simulink model "Ex6_2"  (Simulink 6.0)
settings: Solver=FixedStepDiscrete  SolverMode=SingleTasking  StartTime=0.0  StopTime=Ts*10  FixedStep=Ts  RelTol=1e-3  AbsTol=1e-6
values from neighbouring files (symbols this model uses):
  Ampl = 10^(Amp_dB/20)    (= 0.758577575029)    [Ex6_4Launch.m]
  finrad = Fin*2*pi    (= 28141.7979422)    [Ex6_4Launch.m]
  MultiBit = 1    [Ex6_4Launch.m]
  Ncomp = 1    [Ex6_4Launch.m]
  QuantSat = 0    [Ex6_4Launch.m]
  SatFirst = 1    [Ex6_4Launch.m]
  SatQuant = 0    [Ex6_4Launch.m]
  SatSecond = 1    [Ex6_4Launch.m]
  Ts = 1/Fs    (= 3.54308390023e-07)    [Ex6_4Launch.m]
  VrefN = -1    [Ex6_4Launch.m]
  VrefP = 1    [Ex6_4Launch.m]
  Vsat1 = 1.85    [Ex6_4Launch.m]
  Vsat2 = 2.5    [Ex6_4Launch.m]
undefined symbols (not defined in the file or in its folder): Quantiz
settings Model: Creator=francomaloberti  LastModifiedBy=Cri  ExtModeAutoUpdateStatusClock=off
settings DataIOCC: LimitDataPoints=off  SignalLoggingName=sigsOut
settings OptimizationCC: BooleanDataType=off  InlineInvariantSignals=off
settings DebuggingCC: SolverPrmCheckMsg=none
settings HardwareCC: TargetUnknown=on

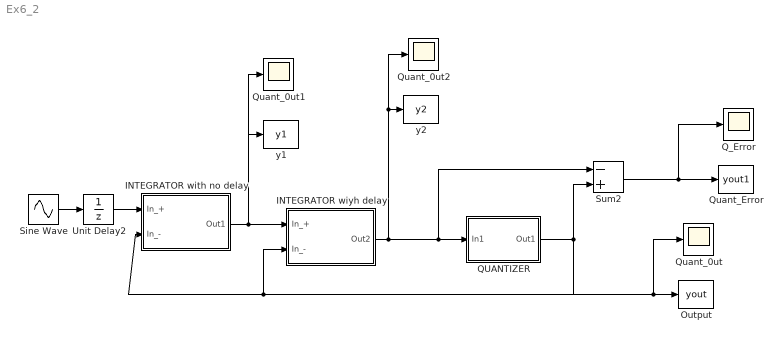
== system Ex6_2 ==
  INTEGRATOR with no delay : Subsystem
      mask Display:
      | patch([10 40 10 10], [0 20 40 0],[0 1 1])
      | plot([10 40 10 10], [0 20 40 0])
      | plot([0 10], [8 8])
      | plot([0 10], [28 28])
      | dpoly([1], [1 -1], 'z-')
      | port_label('input', 1, '+')
      | port_label('input', 2, '-')
  INTEGRATOR wiyh delay : Subsystem
      mask Display:
      | patch([10 40 10 10], [0 20 40 0],[1 0 1])
      | plot([10 40 10 10], [0 20 40 0])
      | plot([0 10], [8 8])
      | plot([0 10], [28 28])
      | dpoly([0 1], [1 -1], 'z-')
      | port_label('input', 1, '+')
      | port_label('input', 2, '-')
  Output : ToWorkspace  VariableName=yout  SampleTime=-1  SaveFormat=Array
  QUANTIZER : Subsystem
      mask Display:
      | plot([0 5 5 10 10 15 15], [0 0 5 5 10 10 15])
      | plot([25 30 30 35], [0 0 15 15])
      | disp('  or')
  Q_Error : Scope
      settings: SaveName=ScopeData2
  Quant_0ut : Scope
  Quant_0ut1 : Scope
  Quant_0ut2 : Scope
      settings: SaveName=ScopeData3
  Quant_Error : ToWorkspace  VariableName=yout1  SampleTime=-1  SaveFormat=Array
  Sine Wave : Sin  Amplitude=Ampl  Frequency=finrad  SampleTime=0
  Sum2 : Sum  Inputs=-+  SaturateOnIntegerOverflow=on  InputSameDT=on
  Unit Delay2 : UnitDelay  SampleTime=Ts
  y1 : ToWorkspace  VariableName=y1  SampleTime=-1  SaveFormat=Array
  y2 : ToWorkspace  VariableName=y2  SampleTime=-1  SaveFormat=Array
  wires:
  Sine Wave/1 -> Unit Delay2/1
  Unit Delay2/1 -> INTEGRATOR with no delay/1(In_+)
  INTEGRATOR wiyh delay/1(Out2) -> QUANTIZER/1(In1), Sum2/1, y2/1, Quant_0ut2/1
  INTEGRATOR with no delay/1(Out1) -> INTEGRATOR wiyh delay/1(In_+), y1/1, Quant_0ut1/1
  QUANTIZER/1(Out1) -> Sum2/2, INTEGRATOR wiyh delay/2(In_-), INTEGRATOR with no delay/2(In_-), Output/1, Quant_0ut/1
  Sum2/1 -> Q_Error/1, Quant_Error/1

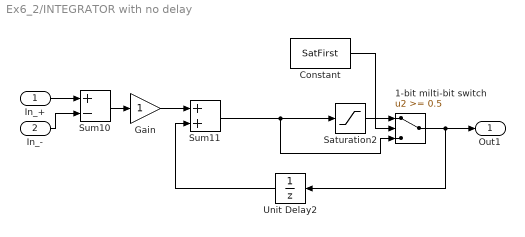
== system Ex6_2/INTEGRATOR with no delay ==
  In_+ : Inport  Port=1  LatchInput=off
  In_- : Inport  Port=2  LatchInput=off
  1-bit milti-bit switch : Switch  Threshold=0.5
  Constant : Constant  Value=SatFirst
  Gain : Gain  SaturateOnIntegerOverflow=on
  Saturation2 : Saturate  UpperLimit=Vsat1  LowerLimit=-Vsat1
  Sum10 : Sum  Inputs=+-  SaturateOnIntegerOverflow=on  InputSameDT=on
  Sum11 : Sum  SaturateOnIntegerOverflow=on  InputSameDT=on
  Unit Delay2 : UnitDelay  Orientation=left  SampleTime=Ts
  Out1 : Outport
  wires:
  Constant/1 -> 1-bit milti-bit switch/2
  1-bit milti-bit switch/1 -> Out1/1, Unit Delay2/1
  Saturation2/1 -> 1-bit milti-bit switch/1
  In_+/1 -> Sum10/1
  In_-/1 -> Sum10/2
  Sum11/1 -> 1-bit milti-bit switch/3, Saturation2/1
  Sum10/1 -> Gain/1
  Gain/1 -> Sum11/1
  Unit Delay2/1 -> Sum11/2

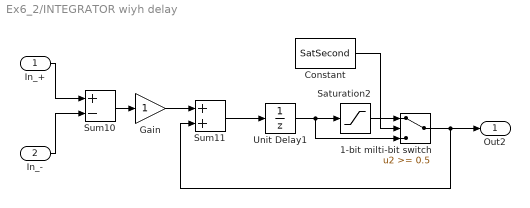
== system Ex6_2/INTEGRATOR wiyh delay ==
  In_+ : Inport  Port=1  LatchInput=off
  In_- : Inport  Port=2  LatchInput=off
  1-bit milti-bit switch : Switch  Threshold=0.5
  Constant : Constant  Value=SatSecond
  Gain : Gain  SaturateOnIntegerOverflow=on
  Saturation2 : Saturate  UpperLimit=Vsat2  LowerLimit=-Vsat2
  Sum10 : Sum  Inputs=+-  SaturateOnIntegerOverflow=on  InputSameDT=on
  Sum11 : Sum  SaturateOnIntegerOverflow=on  InputSameDT=on
  Unit Delay1 : UnitDelay  SampleTime=Ts
  Out2 : Outport
  wires:
  Gain/1 -> Sum11/1
  Sum10/1 -> Gain/1
  Sum11/1 -> Unit Delay1/1
  In_-/1 -> Sum10/2
  In_+/1 -> Sum10/1
  Unit Delay1/1 -> Saturation2/1, 1-bit milti-bit switch/3
  Saturation2/1 -> 1-bit milti-bit switch/1
  1-bit milti-bit switch/1 -> Out2/1, Sum11/2
  Constant/1 -> 1-bit milti-bit switch/2

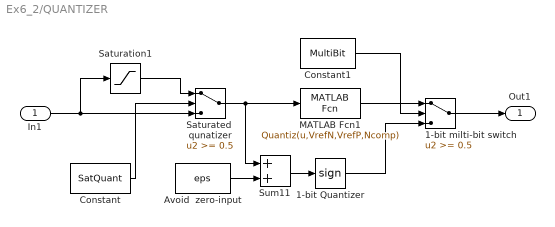
== system Ex6_2/QUANTIZER ==
  In1 : Inport  Port=1  LatchInput=off
  1-bit Quantizer : Signum
  1-bit milti-bit switch : Switch  Threshold=0.5
  Avoid  zero-input : Constant  Value=eps
  Constant : Constant  Value=SatQuant
  Constant1 : Constant  Value=MultiBit
  MATLAB Fcn1 : MATLABFcn  MATLABFcn=Quantiz(u,VrefN,VrefP,Ncomp)
  Saturated  qunatizer : Switch  Threshold=0.5
  Saturation1 : Saturate  UpperLimit=QuantSat  LowerLimit=-QuantSat
  Sum11 : Sum  SaturateOnIntegerOverflow=on  InputSameDT=on
  Out1 : Outport
  wires:
  In1/1 -> Saturated  qunatizer/3, Saturation1/1
  Saturation1/1 -> Saturated  qunatizer/1
  Saturated  qunatizer/1 -> MATLAB Fcn1/1, Sum11/1
  Constant/1 -> Saturated  qunatizer/2
  MATLAB Fcn1/1 -> 1-bit milti-bit switch/1
  1-bit Quantizer/1 -> 1-bit milti-bit switch/3
  Constant1/1 -> 1-bit milti-bit switch/2
  1-bit milti-bit switch/1 -> Out1/1
  Sum11/1 -> 1-bit Quantizer/1
  Avoid  zero-input/1 -> Sum11/2
